simulink model "condExecSample01"  (Simulink 7.8)
settings: Solver=FixedStepDiscrete  StartTime=0.0  StopTime=10.0  FixedStep=Auto  RelTol=1e-3
settings Model: Creator=itoy  LastModifiedBy=itoy
settings DataIOCC: LimitDataPoints=off  SaveFormat=StructureWithTime  SaveOutput=off  SaveTime=off
settings OptimizationCC: ConditionallyExecuteInputs=off  InlineParams=on  OptimizeModelRefInitCode=on  LifeSpan=1
settings DebuggingCC: StrictBusMsg=Warning
settings RTWCC: SystemTargetFile=ert.tlc  GenCodeOnly=on  TemplateMakefile=ert_default_tmf  Description=Real-Time Workshop Embedded Coder  GenerateReport=on  ProcessScript=ert_make_rtw_hook  IncludeHyperlinkInReport=on  LaunchReport=on  GenerateTraceInfo=on  GenerateTraceReport=on  GenerateTraceReportSl=on  GenerateTraceReportSf=on  GenerateTraceReportEml=on
settings CodeAppCC: IgnoreCustomStorageClasses=off
settings ERTTargetCC: MultiwordLength=2048  GenerateSampleERTMain=on  ERTCustomFileTemplate=example_file_process.tlc  ConvertIfToSwitch=off  SuppressUnreachableDefaultCases=off
settings ConfigComp: Description=Design Verifier Custom Configuration Component  DVMaxTestCaseSteps=500  DVTestSuiteOptimization=CombinedObjectives (Nonlinear Extended)

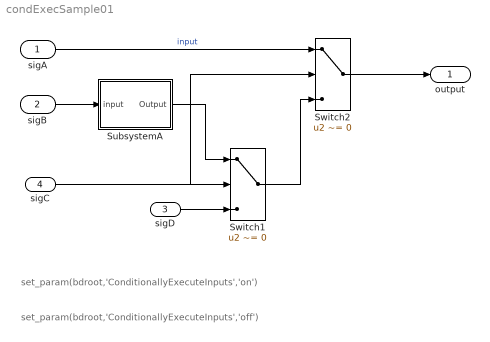
== system condExecSample01 ==
  note: set_param(bdroot,'ConditionallyExecuteInputs','on')
  note: set_param(bdroot,'ConditionallyExecuteInputs','off')
  sigA : Inport  OutDataTypeStr=double  PortDimensions=1
  sigB : Inport  Port=2  OutDataTypeStr=double  PortDimensions=1
  sigD : Inport  Port=3
  sigC : Inport  Port=4  OutDataTypeStr=boolean
  SubsystemA : Subsystem  TreatAsAtomicUnit=on
  Switch1 : Switch  Criteria=u2 ~= 0
      settings: AttributesFormatString=%<Criteria>
  Switch2 : Switch  Criteria=u2 ~= 0
      settings: AttributesFormatString=%<Criteria>
  output : Outport
  wires:
  Switch2/1 -> output/1
  sigD/1 -> Switch1/3
  sigC/1 -> Switch1/2, Switch2/2
  sigA/1 -> Switch2/1  "input"
  Switch1/1 -> Switch2/3
  SubsystemA/1(Output) -> Switch1/1
  sigB/1 -> SubsystemA/1(input)

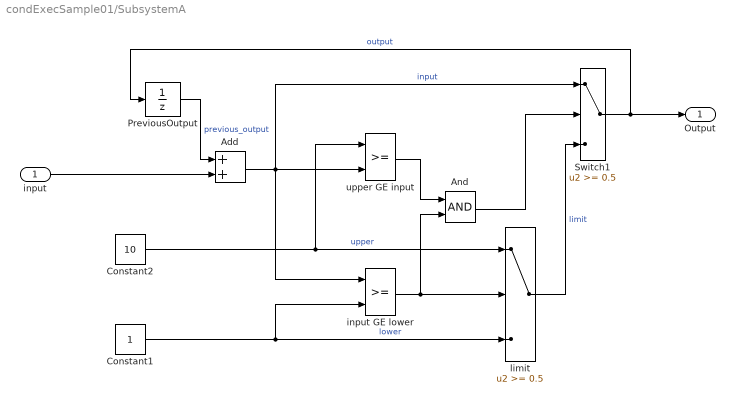
== system condExecSample01/SubsystemA ==
  input : Inport
  " input GE lower" : RelationalOperator  Priority=1  InputSameDT=on
      settings: AttributesFormatString=\n
  " limit" : Switch  Threshold=0.5  SaturateOnIntegerOverflow=on  InputSameDT=on
  Add : Sum
  And : Logic
  Constant1 : Constant
  Constant2 : Constant  Value=10
  PreviousOutput : UnitDelay  SampleTime=-1
  Switch1 : Switch  Threshold=0.5  SaturateOnIntegerOverflow=on  InputSameDT=on
  upper GE input : RelationalOperator  Priority=0  InputSameDT=on
      settings: AttributesFormatString=\n
  Output : Outport
  wires:
  Switch1/1 -> PreviousOutput/1, Output/1  "output"
  " limit"/1 -> Switch1/3  "limit"
  upper GE input/1 -> And/1
  Constant2/1 -> upper GE input/1, " limit"/1  "upper"
  " input GE lower"/1 -> " limit"/2, And/2
  And/1 -> Switch1/2
  Add/1 -> Switch1/1, " input GE lower"/1, upper GE input/2  "input"
  PreviousOutput/1 -> Add/1  "previous_output"
  Constant1/1 -> " input GE lower"/2, " limit"/3  "lower"
  input/1 -> Add/2
